simulink library "netZeroSpoolingControllerEllipse"  (R2018b)
settings: Solver=VariableStepAuto  StartTime=0.0  StopTime=10.0  RelTol=1e-3
undefined symbols (not defined in the file or in its folder): pathCtrl, SPOOLINGCONTROLLER
libraries: simulink x5, runningAvg_ul x2, dspsigops x1, filteredPIDController_ul x1
settings Model: Creator=jcreed2  LastModifiedBy=jcreed2

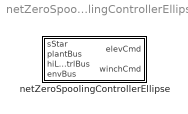
== system netZeroSpoolingControllerEllipse ==
  netZeroSpoolingControllerEllipse : Subsystem  VariantControl=strcmpi(SPOOLINGCONTROLLER,'netZeroSpoolingControllerEllipse')  mask{sigmaVecInit=[.5 .25], reelInDefl=pathCtrl.elevatorReelInDef.Value, reelOutDefl=0}
      mask prompts: sigmaVecInit "Init Spooling Param Vec [center width]"; reelInDefl "Reel In Elevator Deflection [deg]"; reelOutDefl "Reel Out Elevator Deflection [deg]"

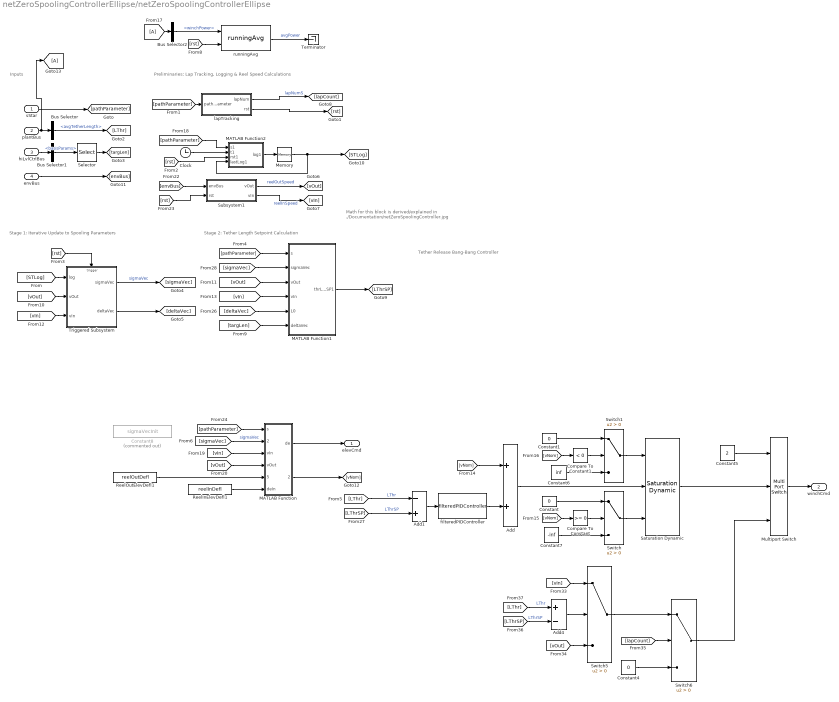
== system netZeroSpoolingControllerEllipse/netZeroSpoolingControllerEllipse ==
  note: Tether Release Bang-Bang Controller
  note: Inputs
  note: Stage 1: Iterative Update to Spooling Parameters
  note: Preliminaries: Lap Tracking, Logging & Reel Speed Calculations
  note: Math for this block is derived/explained in
      | ./Documentation/netZeroSpoolingController.jpg
  note: Stage 2: Tether Length Setpoint Calculation
  "sStar " : Inport
  plantBus : Inport  Port=2  OutDataTypeStr=Bus: plantBus
  hiLvlCtrlBus : Inport  Port=3  OutDataTypeStr=Bus: hiLvlCtrlBus
  envBus : Inport  Port=4  OutDataTypeStr=Bus: envBus
  Add : Sum
  Add1 : Sum  Inputs=-+
  Add4 : Sum  Inputs=+-
  Bus Selector : BusSelector  OutputSignals=avgTetherLength
  Bus Selector1 : BusSelector  OutputSignals=basisParams
  Bus Selector2 : BusSelector  OutputSignals=winchPower
  Clock : Clock
  Compare To Constant : simulink/Logic and Bit Operations/Compare To Constant  relop=>=  const=0  OutDataTypeStr=boolean
  Compare To Constant1 : simulink/Logic and Bit Operations/Compare To Constant  relop=<  const=0  OutDataTypeStr=boolean
  Constant : Constant  Value=0
  Constant1 : Constant  Value=0
  Constant4 : Constant  Value=0
  Constant5 : Constant  Value=2
  Constant6 : Constant  Value=inf
  Constant7 : Constant  Value=-inf
  Constant8 : Constant  Commented=on  Value=sigmaVecInit
  MATLAB Function : MATLAB Function  TreatAsAtomicUnit=on
  MATLAB Function1 : MATLAB Function  TreatAsAtomicUnit=on
  MATLAB Function2 : MATLAB Function  TreatAsAtomicUnit=on
  Memory : Memory
  Multiport Switch : MultiPortSwitch  Inputs=2
  ReelInElevDefl1 : Constant  Value=reelInDefl
  ReelOutElevDefl1 : Constant  Value=reelOutDefl
  Saturation Dynamic : simulink/Discontinuities/Saturation Dynamic  OutMin=[]  OutMax=[]  OutDataTypeStr=Inherit: Same as second input  OutDataType=fixdt(1, 16)  OutScaling=2^-10  DoSatur=off
  Selector : Selector  InputPortWidth=5  IndexOptions=Index vector (dialog)  Indices=5  OutputSizes=1
  Subsystem1 : Subsystem
  Switch{,1,5..6} (4 alike) : Switch  Criteria=u2 > Threshold
  Terminator : Terminator
  Triggered Subsystem : Subsystem  TreatAsAtomicUnit=on
  filteredPIDController : filteredPIDController_ul/filteredPIDController  kp=.1  ki=0  kd=0  Value=0
  lapTracking : Subsystem
  runningAvg : runningAvg_ul/runningAvg  SystemSampleTime=-1
  elevCmd : Outport
  "winchCmd " : Outport  Port=2
  wires:
  Bus Selector1/1 -> Selector/1  "<basisParams>"
  Compare To Constant1/1 -> Switch1/2
  Bus Selector/1 -> [LThr]  "<avgTetherLength>"
  [pathParameter] -> MATLAB Function2/1(s1)
  Constant1/1 -> Switch1/1
  [vIn] -> MATLAB Function/3(vIn)
  Selector/1 -> [targLen]
  [envBus] -> Subsystem1/1(envBus)
  lapTracking/1(lapNum) -> [lapCount]  "lapNumS"
  [STLog] -> Triggered Subsystem/1(log)
  Compare To Constant/1 -> Switch/2
  MATLAB Function/2(vNominal) -> [vNom]
  ReelOutElevDefl1/1 -> MATLAB Function/5(deOut)
  Switch1/1 -> Saturation Dynamic/1
  [LThrSP] -> Add1/2  "LThrSP"
  Constant6/1 -> Switch1/3
  Constant7/1 -> Switch/3
  plantBus/1 -> Bus Selector/1, [A]
  Triggered Subsystem/2(deltaVec) -> [deltaVec]
  [LThr] -> Add1/1  "LThr"
  Switch6/1 -> Multiport Switch/3
  Memory/1 -> MATLAB Function2/4(lastLog1), [STLog]
  lapTracking/2(rst) -> [rst]
  [A] -> Bus Selector2/1
  [vOut] -> Switch5/3
  Constant4/1 -> Switch6/3
  [rst] -> runningAvg/2
  [lapCount] -> Switch6/2
  Multiport Switch/1 -> "winchCmd "/1
  [vIn] -> Switch5/1
  [vNom] -> Compare To Constant1/1
  [sigmaVec] -> MATLAB Function/2(sigmaVec)  "sigmaVec"
  hiLvlCtrlBus/1 -> Bus Selector1/1
  MATLAB Function/1(de) -> elevCmd/1
  Switch/1 -> Saturation Dynamic/3
  runningAvg/1 -> Terminator/1  "avgPower"
  Triggered Subsystem/1(sigmaVec) -> [sigmaVec]  "sigmaVec"
  Constant5/1 -> Multiport Switch/1
  Add4/1 -> Switch5/2
  Add1/1 -> filteredPIDController/1
  Switch5/1 -> Switch6/1
  Subsystem1/1(vOut) -> [vOut]  "reelOutSpeed"
  [pathParameter] -> lapTracking/1(pathParameter)
  [pathParameter] -> MATLAB Function/1(s)
  Saturation Dynamic/1 -> Multiport Switch/2
  [deltaVec] -> MATLAB Function1/5(L0)
  ReelInElevDefl1/1 -> MATLAB Function/6(deIn)
  filteredPIDController/1 -> Add/2
  [targLen] -> MATLAB Function1/6(deltaVec)
  Constant/1 -> Switch/1
  [sigmaVec] -> MATLAB Function1/2(sigmaVec)
  [vOut] -> MATLAB Function1/3(vOut)
  [vIn] -> MATLAB Function1/4(vIn)
  [pathParameter] -> MATLAB Function1/1(s)
  [rst] -> Subsystem1/2(rst)
  [vIn] -> Triggered Subsystem/3(vIn)
  [vOut] -> Triggered Subsystem/2(vOut)
  "sStar "/1 -> [pathParameter]
  [LThr] -> Add4/1  "LThr"
  envBus/1 -> [envBus]
  Add/1 -> Saturation Dynamic/2
  Subsystem1/2(vIn) -> [vIn]  "reelInSpeed"
  [vNom] -> Add/1
  [rst] -> Triggered Subsystem/Trigger
  Bus Selector2/1 -> runningAvg/1  "<winchPower>"
  [LThrSP] -> Add4/2  "LThrSP"
  MATLAB Function1/1(thrLenSP1) -> [LThrSP]
  [vNom] -> Compare To Constant/1
  [vOut] -> MATLAB Function/4(vOut)
  [rst] -> MATLAB Function2/3(rst1)
  Clock/1 -> MATLAB Function2/2(t1)
  MATLAB Function2/1(log1) -> Memory/1

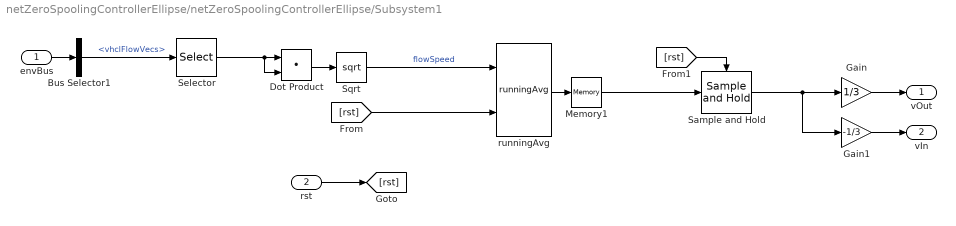
== system netZeroSpoolingControllerEllipse/netZeroSpoolingControllerEllipse/Subsystem1 ==
  envBus : Inport
  rst : Inport  Port=2
  Bus Selector1 : BusSelector  OutputSignals=vhclFlowVecs
  Dot Product : DotProduct  InputSameDT=on  OutDataTypeStr=Inherit: Inherit via internal rule
  Gain : Gain  Gain=1/3
  Gain1 : Gain  Gain=-1/3
  Memory1 : Memory
  Sample and Hold : dspsigops/Sample and Hold  trig=Rising edge  initCond=0  latchinput=off
  Selector : Selector  NumberOfDimensions=2  InputPortWidth=3  IndexOptions=Select all,Index vector (dialog)  Indices=[1 3],5  OutputSizes=1,1
  Sqrt : Sqrt  SaturateOnIntegerOverflow=on
  runningAvg : runningAvg_ul/runningAvg  SystemSampleTime=-1
  vOut : Outport
  vIn : Outport  Port=2
  wires:
  Selector/1 -> Dot Product/2, Dot Product/1
  Dot Product/1 -> Sqrt/1
  runningAvg/1 -> Memory1/1
  [rst] -> Sample and Hold/Trigger
  Gain/1 -> vOut/1
  Gain1/1 -> vIn/1
  Sample and Hold/1 -> Gain1/1, Gain/1
  envBus/1 -> Bus Selector1/1
  Sqrt/1 -> runningAvg/1  "flowSpeed"
  Memory1/1 -> Sample and Hold/1
  [rst] -> runningAvg/2
  Bus Selector1/1 -> Selector/1  "<vhclFlowVecs>"
  rst/1 -> [rst]

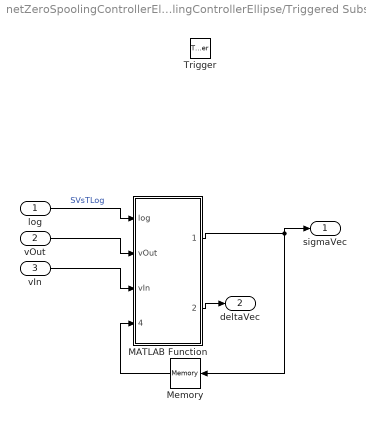
== system netZeroSpoolingControllerEllipse/netZeroSpoolingControllerEllipse/Triggered Subsystem ==
  log : Inport
  vOut : Inport  Port=2
  vIn : Inport  Port=3
  Trigger : TriggerPort  VariantControl=Variant
  MATLAB Function : MATLAB Function  TreatAsAtomicUnit=on
  Memory : Memory  InitialCondition=sigmaVecInit  InheritSampleTime=on
  sigmaVec : Outport  InitialOutput=sigmaVecInit
  deltaVec : Outport  Port=2  InitialOutput="[0.0136    0.0097    0.0198    0.0152    0.0208]"
  wires:
  log/1 -> MATLAB Function/1(log)  "SVsTLog"
  vOut/1 -> MATLAB Function/2(vOut)
  vIn/1 -> MATLAB Function/3(vIn)
  MATLAB Function/2(deltaVec) -> deltaVec/1
  MATLAB Function/1(sigmaVec) -> Memory/1, sigmaVec/1
  Memory/1 -> MATLAB Function/4(sigmaVecInit)

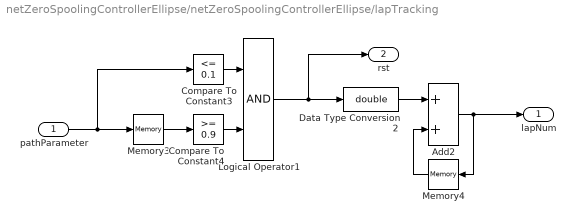
== system netZeroSpoolingControllerEllipse/netZeroSpoolingControllerEllipse/lapTracking ==
  pathParameter : Inport
  Add2 : Sum
  Compare To Constant3 : simulink/Logic and Bit Operations/Compare To Constant  relop=<=  const=0.1  OutDataTypeStr=boolean
  Compare To Constant4 : simulink/Logic and Bit Operations/Compare To Constant  relop=>=  const=0.9  OutDataTypeStr=boolean
  Data Type Conversion2 : DataTypeConversion  OutDataTypeStr=double
  Logical Operator1 : Logic  AllPortsSameDT=off  OutDataTypeStr=boolean
  Memory3 : Memory
  Memory4 : Memory
  lapNum : Outport
  rst : Outport  Port=2
  wires:
  Compare To Constant3/1 -> Logical Operator1/1
  pathParameter/1 -> Compare To Constant3/1, Memory3/1
  Compare To Constant4/1 -> Logical Operator1/2
  Memory3/1 -> Compare To Constant4/1
  Logical Operator1/1 -> rst/1, Data Type Conversion2/1
  Data Type Conversion2/1 -> Add2/1
  Memory4/1 -> Add2/2
  Add2/1 -> lapNum/1, Memory4/1

== matlab function netZeroSpoolingControllerEllipse/MATLAB Function1 ==
  data: s input; thrLenSP1 output; sigmaVec input; vOut input; vIn input; L0 input; deltaVec input
function thrLenSP1  = fcn(s,sigmaVec,vOut,vIn,L0,deltaVec)

thrLenSP1 = LThrInt1(s,sigmaVec,vOut,vIn,L0,deltaVec);

end

== matlab function netZeroSpoolingControllerEllipse/Triggered Subsystem/MATLAB Function ==
  data: log input; sigmaVec output; vOut input; vIn input; sigmaVecInit input; deltaVec output
function [sigmaVec,deltaVec] = fcn(log,vOut,vIn,sigmaVecInit)

sc = sigmaVecInit(1);
sw = sigmaVecInit(2);
sigmaVec = sigmaVecInit;

cleanLog = [0 0;...
    log(and(log(:,1)~=0,log(:,2)~=0),:)];
 
% Extract regions
r1 = cleanLog(and(cleanLog(:,1)>=0        ,cleanLog(:,1)<sc-sw),:);
r2 = cleanLog(and(cleanLog(:,1)>=sc-sw    ,cleanLog(:,1)<sc+sw),:);
r3 = cleanLog(and(cleanLog(:,1)>=sc+sw    ,cleanLog(:,1)<=1),:);


% Calculate average numerical derivative in each region ds/dt
ds1 = mean(diff(r1(:,1))./diff(r1(:,2)));
ds2 = mean(diff(r2(:,1))./diff(r2(:,2)));
ds3 = mean(diff(r3(:,1))./diff(r3(:,2)));


deltaVec = [ds1 ds2 ds3]';

dsInv = diag([1/ds1 1/ds2 1/ds3 ]);

V = diag([vOut vIn vOut ]);

Delta = eye(3);
Delta(2,1) = -1;
Delta(3,2) = -1;


A  = [ 0  0 1]';
B1 = [ 1  1  0]';
B2 = [-1  1  0]';

c1 = ones(1,3)*V*dsInv*Delta*(A+B1*sc);
c2 = ones(1,3)*V*dsInv*Delta*B2;
sw = min([max([-c1/c2 0]) sc]); % 0<=sw<=sc
sigmaVec(2) = sw;

% Note: the following code alternates between updating sc and sw.
% After a bit of testing, I found that the update on sc was really screwing
% things up.  Not sure why that is at the moment, but it's kind of
% irrelevant since the update on sw alone works well enough.  Moving on.
% -MC

% Alternate updaing sc and sw each lap
% if mod(round(lapNum),2) % Odd lap number
    % Case 1, sc fixed, update sw
%     sigmaVec(1) = sc;
%     c1 = ones(1,5)*V*dsInv*Delta*(A+B1*sc);
%     c2 = ones(1,5)*V*dsInv*Delta*B2;
%     sw = min([max([-c1/c2 0]) sc]); % 0<=sw<=0.25
% else % Even lap number
%     % Case 2, sw fixed, update sc
% %     sigmaVec(2) = sw;
%     c1 = ones(1,5)*V*dsInv*Delta*(A+B2*sw);
%     c2 = ones(1,5)*V*dsInv*Delta*B1;
%     sc = min([max([-c1/c2 sw]) 0.5-sw]);
% end

% sigmaVec(1) = sc;
% sigmaVec(2) = sw;

== matlab function netZeroSpoolingControllerEllipse/MATLAB Function ==
  data: s input; de output; sigmaVec input; vIn input; vOut input; deOut input; deIn input; vNominal output
function [de,vNominal] = fcn(s,sigmaVec,vIn,vOut,deOut,deIn)
vNominal = vOut;
de = deOut;

sc = sigmaVec(1);
sw = sigmaVec(2);

if s>=sc-sw && s<=sc+sw
    vNominal = vIn;
    de = deIn;
    return
end


end

== matlab function netZeroSpoolingControllerEllipse/MATLAB Function2 ==
  data: s1 input; log1 output; t1 input; rst1 input; lastLog1 input
function log1  = fcn(s1,t1,rst1,lastLog1)
% function that logs the path position and time into a matrix
% [pathPosition,t]
if rst1
    lastLog1 = nan(1000,2);
end
log1 = lastLog1;
idx = min([max([round(s1*1000),1]),1000]);
log1(idx,1) = s1;
log1(idx,2) = t1;
end
